simulink model "SimpleLegTest"  (R2014a)
settings: Solver=ode3  SolverMode=SingleTasking  StartTime=0.0  StopTime=10.0  RelTol=1e-3
libraries: arduinolib x5
settings Model: ExtModeTrigDuration=2  Creator=beaverl  LastModifiedBy=beaverl
settings OptimizationCC: OptimizeModelRefInitCode=on  LifeSpan=1
settings DebuggingCC: UnderspecifiedInitializationDetection=Classic  SolverPrmCheckMsg=none
settings HardwareCC: ProdBitPerInt=16  ProdBitPerPointer=8  ProdIntDivRoundTo=Zero  ProdEndianess=LittleEndian  ProdWordSize=8  ProdHWDeviceType=Atmel->AVR
settings RTWCC: SystemTargetFile=realtime.tlc  GenerateMakefile=off  TemplateMakefile=realtime.tmf  Description=Run on Target Hardware  RTWVerbose=off  ProcessScript=realtime_make_rtw_hook
settings STFCustomTargetCC: TargetLibSuffix=.a  GenerateSampleERTMain=on  ConcurrentExecutionCompliant=off  GeneratePreprocessorConditionals=Use local settings  ERTCustomFileBanners=on  SupportNonInlinedSFcns=off  SupportVariableSizeSignals=on  MATLABClassNameForMDSCustomization=Simulink.SoftwareTarget.ERTCustomization  GRTInterface=off  SystemTargetFile=realtime.tlc
settings ERTTargetCC: CombineOutputUpdateFcns=off  SupportContinuousTime=on  SupportVariableSizeSignals=on  ExtModeTransport=3  ExtModeMexFile=ext_serial_win32_comm  ExtModeMexArgs=0 1 9600  ERTSrcFileBannerTemplate=realtime_code_template.cgt  ERTHdrFileBannerTemplate=realtime_code_template.cgt  ERTDataSrcFileTemplate=realtime_code_template.cgt  ERTDataHdrFileTemplate=realtime_code_template.cgt  ERTCustomFileTemplate=realtime_file_process.tlc

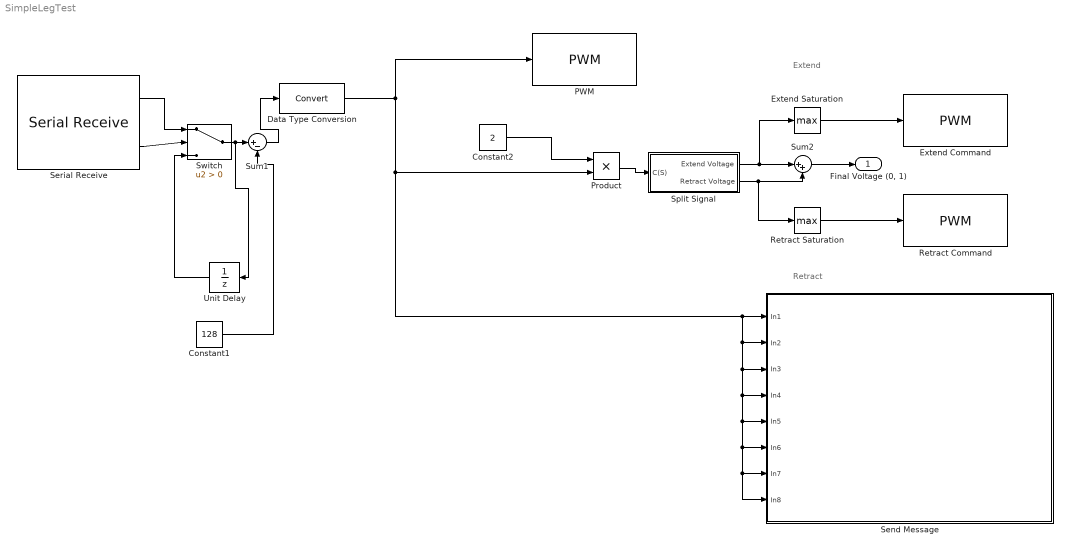
== system SimpleLegTest ==
  note: Retract
  note: Extend
  Constant1 : Constant  Value=128
  Constant2 : Constant  Value=2
  Data Type Conversion : DataTypeConversion  SaturateOnIntegerOverflow=on
  Extend Command : arduinolib/PWM  pinNumber=2
  Extend Saturation : MinMax  Function=max  OutMin=[0]  OutMax=[255]  OutDataTypeStr=int16  SaturateOnIntegerOverflow=on
  PWM : arduinolib/PWM  pinNumber=5
  Product : Product
  Retract Command : arduinolib/PWM  pinNumber=4
  Retract Saturation : MinMax  Function=max  OutMin=[0]  OutMax=[255]  OutDataTypeStr=int16  SaturateOnIntegerOverflow=on
  Send Message : Subsystem
  Serial Receive : arduinolib/Serial Receive  portNumber=1  showOutStatus=on  sampleTime=.02
  Split Signal : Subsystem
  Sum1 : Sum  Inputs=|+-
  Sum2 : Sum  Inputs=|++
  Switch : Switch  Criteria=u2 > Threshold
  Unit Delay : UnitDelay  SampleTime=-1
  "Final Voltage (0, 1)" : Outport
  wires:
  Serial Receive/2 -> Switch/2
  Serial Receive/1 -> Switch/1
  Split Signal/1(Extend Voltage) -> Extend Saturation/1, Sum2/1
  Sum2/1 -> "Final Voltage (0, 1)"/1
  Split Signal/2(Retract Voltage) -> Retract Saturation/1, Sum2/2
  Extend Saturation/1 -> Extend Command/1
  Retract Saturation/1 -> Retract Command/1
  Product/1 -> Split Signal/1(C(S))
  Data Type Conversion/1 -> Send Message/8(In8), Send Message/7(In7), Send Message/6(In6), Send Message/5(In5), Send Message/4(In4), Send Message/3(In3), Send Message/2(In2), Send Message/1(In1), Product/2, PWM/1
  Constant2/1 -> Product/1
  Constant1/1 -> Sum1/2
  Switch/1 -> Unit Delay/1, Sum1/1
  Sum1/1 -> Data Type Conversion/1
  Unit Delay/1 -> Switch/3

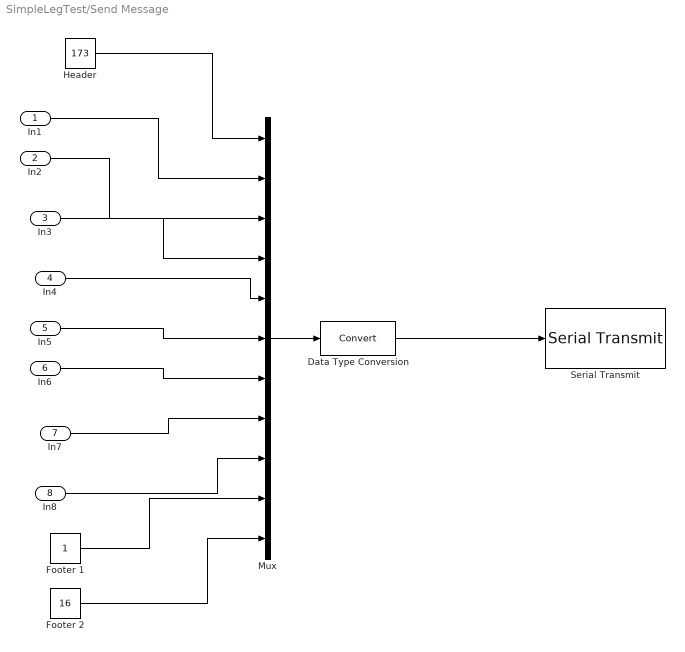
== system SimpleLegTest/Send Message ==
  In1 : Inport
  In2 : Inport  Port=2
  In3 : Inport  Port=3
  In4 : Inport  Port=4
  In5 : Inport  Port=5
  In6 : Inport  Port=6
  In7 : Inport  Port=7
  In8 : Inport  Port=8
  Data Type Conversion : DataTypeConversion  SaturateOnIntegerOverflow=on
  Footer 1 : Constant
  Footer 2 : Constant  Value=16
  Header : Constant  Value=173
  Mux : Mux  Inputs=11
  Serial Transmit : arduinolib/Serial Transmit  portNumber=1
  wires:
  In1/1 -> Mux/2
  In2/1 -> Mux/3
  In3/1 -> Mux/4
  In4/1 -> Mux/5
  In5/1 -> Mux/6
  In6/1 -> Mux/7
  In7/1 -> Mux/8
  In8/1 -> Mux/9
  Header/1 -> Mux/1
  Footer 1/1 -> Mux/10
  Footer 2/1 -> Mux/11
  Mux/1 -> Data Type Conversion/1
  Data Type Conversion/1 -> Serial Transmit/1

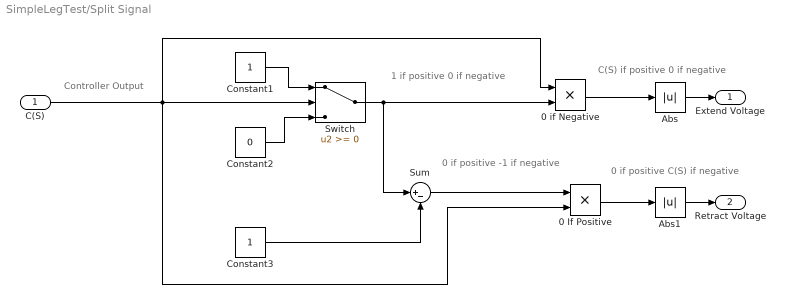
== system SimpleLegTest/Split Signal ==
  note: Controller Output
  note: 0 if positive
      | C(S) if negative
  note: C(S) if positive
      | 0 if negative
  note: 0 if positive
      | -1 if negative
  note: 1 if positive
      | 0 if negative
  C(S) : Inport
  0 If Positive : Product
  0 if Negative : Product
  Abs : Abs
  Abs1 : Abs
  Constant1 : Constant
  Constant2 : Constant  Value=0
  Constant3 : Constant
  Sum : Sum  Inputs=|+-
  Switch : Switch
  Extend Voltage : Outport
  Retract Voltage : Outport  Port=2
  wires:
  Constant1/1 -> Switch/1
  Constant2/1 -> Switch/3
  Switch/1 -> 0 if Negative/2, Sum/1
  Constant3/1 -> Sum/2
  0 If Positive/1 -> Abs1/1
  C(S)/1 -> 0 If Positive/2, 0 if Negative/1, Switch/2
  Sum/1 -> 0 If Positive/1
  0 if Negative/1 -> Abs/1
  Abs/1 -> Extend Voltage/1
  Abs1/1 -> Retract Voltage/1
